simulink model "QCar2_Virtual_Car3"  (R2023a)
settings: Solver=ode1  StartTime=0.0  StopTime=inf  FixedStep=cameraStepSize/10  RelTol=1e-3  EnableMultiTasking=on
PreLoadFcn:
  | QCarSetup
values from neighbouring files (symbols this model uses):
  cameraStepSize = 3e-2    (= 0.03)    [QCarSetup.m]
  path_x = [0.826 0.836 0.846 0.856 0.866 0.876 0.886 0.896 0.906 0.916 0.926 0.936 ... (740 elements, 740x1)]    [SDTS_Paths_6_2023.mat]
  path_x2 = [-0.614 -0.604 -0.594 -0.584 -0.574 -0.564 -0.554 -0.544 -0.534 -0.524 -0.514 -0.504 ... (1090 elements, 1090x1)]    [SDTS_Paths_6_2023.mat]
  path_x3 = [-0.614 -0.603821428571 -0.593642857143 -0.583464285714 -0.573285714286 -0.563107142857 -0.552928571429 -0.54275 -0.532571428571 -0.522392857143 -0.512214285714 -0.502035714286 ... (714 elements, 714x1)]    [SDTS_Paths_6_2023.mat]
  path_x4 = [-0.614 -0.604 -0.594 -0.584 -0.574 -0.564 -0.554 -0.544 -0.534 -0.524 -0.514 -0.504 ... (1761 elements, 1761x1)]    [SDTS_Paths_6_2023.mat]
  path_x5 = [1.436 1.42588571429 1.41577142857 1.40565714286 1.39554285714 1.38542857143 1.37531428571 1.3652 1.35508571429 1.34497142857 1.33485714286 1.32474285714 ... (574 elements, 574x1)]    [SDTS_Paths_6_2023.mat]
  path_x6 = [1.436 1.42588571429 1.41577142857 1.40565714286 1.39554285714 1.38542857143 1.37531428571 1.3652 1.35508571429 1.34497142857 1.33485714286 1.32474285714 ... (1288 elements, 1288x1)]    [SDTS_Paths_6_2023.mat]
  path_y = [-1.0887 -1.0887 -1.0887 -1.0887 -1.0887 -1.0887 -1.0887 -1.0887 -1.0887 -1.0887 -1.0887 -1.0887 ... (740 elements, 740x1)]    [SDTS_Paths_6_2023.mat]
  path_y2 = [-1.0887 -1.0887 -1.0887 -1.0887 -1.0887 -1.0887 -1.0887 -1.0887 -1.0887 -1.0887 -1.0887 -1.0887 ... (1090 elements, 1090x1)]    [SDTS_Paths_6_2023.mat]
  path_y3 = [-1.0887 -1.0887 -1.0887 -1.0887 -1.0887 -1.0887 -1.0887 -1.0887 -1.0887 -1.0887 -1.0887 -1.0887 ... (714 elements, 714x1)]    [SDTS_Paths_6_2023.mat]
  path_y4 = [-1.0887 -1.0887 -1.0887 -1.0887 -1.0887 -1.0887 -1.0887 -1.0887 -1.0887 -1.0887 -1.0887 -1.0887 ... (1761 elements, 1761x1)]    [SDTS_Paths_6_2023.mat]
  path_y5 = [-0.8157 -0.8157 -0.8157 -0.8157 -0.8157 -0.8157 -0.8157 -0.8157 -0.8157 -0.8157 -0.8157 -0.8157 ... (574 elements, 574x1)]    [SDTS_Paths_6_2023.mat]
  path_y6 = [-0.8157 -0.8157 -0.8157 -0.8157 -0.8157 -0.8157 -0.8157 -0.8157 -0.8157 -0.8157 -0.8157 -0.8157 ... (1288 elements, 1288x1)]    [SDTS_Paths_6_2023.mat]
undefined symbols (not defined in the file or in its folder): DiscIntNeverNeededParam, gcbh, height, Host, JPEG, left, qc_get_step_size, top, video_display_show, width
libraries: quarc_library x71, simulink_extras x12, simulink x5
(part 3 of 5)

== system QCar2_Virtual_Car3/Speed & Steering Commander/Cross Track Controller ==
  closest point : Inport
  distance : Inport  Port=2
  xy : Inport  Port=3
  Heading : Inport  Port=4
  Cos : Trigonometry  Operator=cos
  Cos1 : Trigonometry
  Cross Product : quarc_library/Math Operations/Vectors/Cross Product
      settings: SourceProductName=QUARC Targets
  Demux : Demux  Outputs=3
  Gain3 : Gain  Gain=2
  Gain6 : Gain  Gain=10
  Integrator : Integrator  LimitOutput=on  UpperSaturationLimit=.25  LowerSaturationLimit=-.25
  Mux : Mux  Inputs=3
  Mux1 : Mux  Inputs=2
  Product3 : Product
  Saturation1 : Saturate  UpperLimit=0.25  LowerLimit=-0.25
  Sign : Signum
  Sum : Sum  Inputs=+-
  Sum2 : Sum
  steering correction : Outport
  wires:
  Sum2/1 -> steering correction/1
  distance/1 -> Product3/2
  Saturation1/1 -> Sum2/2
  Integrator/1 -> Sum2/1
  Product3/1 -> Gain6/1, Gain3/1
  Gain3/1 -> Saturation1/1
  Gain6/1 -> Integrator/1
  Sign/1 -> Product3/1
  Demux/3 -> Sign/1
  Cross Product/1 -> Demux/1
  Mux/1 -> Cross Product/1
  Mux1/1 -> Cross Product/2
  Sum/1 -> Mux1/1
  closest point/1 -> Sum/1
  xy/1 -> Sum/2
  Cos1/1 -> Mux/2
  Cos/1 -> Mux/1
  Heading/1 -> Cos/1, Cos1/1

== system QCar2_Virtual_Car3/Speed & Steering Commander/LiDAR Steering ==
  xy_command : Inport
  xy : Inport  Port=2
  heading : Inport  Port=3
  Direction Vector Generator : Subsystem
  Display1 : Display
      settings: Decimation=100
  Gain1 : Gain
  Radians to Degrees1 : simulink_extras/Transformations/Radians to Degrees
  Steering Commander : MATLAB Function  TreatAsAtomicUnit=on
  distance : Outport
  LiDAR Steering : Outport  Port=2
  wires:
  Steering Commander/1(steering) -> Gain1/1
  heading/1 -> Direction Vector Generator/3(heading)
  xy/1 -> Direction Vector Generator/2(xy)
  Radians to Degrees1/1 -> Display1/1
  Gain1/1 -> LiDAR Steering/1
  Direction Vector Generator/2(aoa) -> Steering Commander/1(aoa), Radians to Degrees1/1
  xy_command/1 -> Direction Vector Generator/1(xy_command)
  Direction Vector Generator/1(distance) -> distance/1

== system QCar2_Virtual_Car3/Speed & Steering Commander/Path Commander ==
  note: Changed the abs and the duration
  path : Inport
  xy : Inport  Port=2
  look_ahead_d : Inport  Port=3
  Constant : Constant  Value=.05
  Constant1 : Constant  Value=.5
  Data Type Conversion : DataTypeConversion  SaturateOnIntegerOverflow=off  RndMeth=Floor
  Display : Display
  "Distance  " : Scope
  Gain : Gain  Gain=[1 1 1 1 1 1]
  Less Than Threshold : Subsystem
  Multiport Switch : MultiPortSwitch  Inputs=6  DiagnosticForDefault=None  SaturateOnIntegerOverflow=off  InputSameDT=off
  Multiport Switch1 : MultiPortSwitch  Inputs=6  DiagnosticForDefault=None  SaturateOnIntegerOverflow=off  InputSameDT=off
  Multiport Switch2 : MultiPortSwitch  Inputs=6  DiagnosticForDefault=None  SaturateOnIntegerOverflow=off  InputSameDT=off
  Mux : Mux  Inputs=6
  Path 1  Look Ahead Generator : Subsystem
  Path 2  Look Ahead Generator : Subsystem
  Path 3  Look Ahead Generator : Subsystem
  Path 4  Look Ahead Generator : Subsystem
  Path 5  Look Ahead Generator : Subsystem
  Path 6  Look Ahead Generator : Subsystem
  xy_cmd : Outport
  Path_Options : Outport  Port=2
  closest point : Outport  Port=3
  distance : Outport  Port=4
  wires:
  Multiport Switch2/1 -> distance/1
  Multiport Switch1/1 -> closest point/1
  Path 6  Look Ahead Generator/2(closest_point) -> Multiport Switch1/7
  Path 5  Look Ahead Generator/2(closest_point) -> Multiport Switch1/6
  Path 4  Look Ahead Generator/2(closest_point) -> Multiport Switch1/5
  Path 3  Look Ahead Generator/2(closest_point) -> Multiport Switch1/4
  Path 2  Look Ahead Generator/2(closest_point) -> Multiport Switch1/3
  Path 1  Look Ahead Generator/2(closest_point) -> Multiport Switch1/2
  Path 6  Look Ahead Generator/3(distance) -> Mux/6, Multiport Switch2/7
  Path 5  Look Ahead Generator/3(distance) -> Mux/5, Multiport Switch2/6
  Path 6  Look Ahead Generator/1(xy_cmd) -> Multiport Switch/7
  Path 5  Look Ahead Generator/1(xy_cmd) -> Multiport Switch/6
  Data Type Conversion/1 -> Gain/1
  Gain/1 -> Path_Options/1
  Less Than Threshold/1(elapsed) -> Display/1, Data Type Conversion/1
  Constant1/1 -> Less Than Threshold/3(Duration)
  Constant/1 -> Less Than Threshold/2(Threshold)
  Mux/1 -> "Distance  "/1, Less Than Threshold/1(Signal)
  Path 4  Look Ahead Generator/3(distance) -> Mux/4, Multiport Switch2/5
  Path 3  Look Ahead Generator/3(distance) -> Mux/3, Multiport Switch2/4
  Path 2  Look Ahead Generator/3(distance) -> Mux/2, Multiport Switch2/3
  Path 1  Look Ahead Generator/3(distance) -> Mux/1, Multiport Switch2/2
  Path 4  Look Ahead Generator/1(xy_cmd) -> Multiport Switch/5
  Path 3  Look Ahead Generator/1(xy_cmd) -> Multiport Switch/4
  Multiport Switch/1 -> xy_cmd/1
  Path 2  Look Ahead Generator/1(xy_cmd) -> Multiport Switch/3
  Path 1  Look Ahead Generator/1(xy_cmd) -> Multiport Switch/2
  path/1 -> Multiport Switch/1, Multiport Switch1/1, Multiport Switch2/1
  xy/1 -> Path 1  Look Ahead Generator/1(xy), Path 2  Look Ahead Generator/1(xy), Path 3  Look Ahead Generator/1(xy), Path 4  Look Ahead Generator/1(xy), Path 5  Look Ahead Generator/1(xy), Path 6  Look Ahead Generator/1(xy)
  look_ahead_d/1 -> Path 1  Look Ahead Generator/2(look_ahead_d), Path 2  Look Ahead Generator/2(look_ahead_d), Path 3  Look Ahead Generator/2(look_ahead_d), Path 4  Look Ahead Generator/2(look_ahead_d), Path 5  Look Ahead Generator/2(look_ahead_d), Path 6  Look Ahead Generator/2(look_ahead_d)

== system QCar2_Virtual_Car3/Speed & Steering Commander/Traffic Zone 1 ==
  note: select the control variable
  xy : Inport
  speed in : Inport  Port=2
  Traffic Light : Inport  Port=3
  AND : Logic  Inputs=4  IconShape=distinctive  AllPortsSameDT=off  OutDataTypeStr=boolean
  Bias : Bias  Bias=-0.3-0.586  SaturateOnIntegerOverflow=off
  Constant13 : Constant  Value=[0.2 -0.7]+[0.586 -0.258]
  Constant14 : Constant  Value=[1 -.3] +[0.586 -0.258]
  Constant3 : Constant  Value=.1
  Demux : Demux  Outputs=2
  Demux1 : Demux  Outputs=2
  Demux2 : Demux  Outputs=2
  Gain : Gain  Gain=1/.7
  Greater Than Threshold : Subsystem
  Less Than Threshold : Subsystem
  MATLAB Function2 : MATLAB Function  TreatAsAtomicUnit=on
  Memory7 : Memory  InitialCondition=1  InheritSampleTime=on  LinearizeMemory=on  LinearizeAsDelay=on
  Saturation : Saturate  UpperLimit=1  LowerLimit=0
  "Speed " : Scope
  Speed Multi : Scope
  Traffic State : Display
  in zone : Display
  Speed Out : Outport
  wires:
  Traffic Light/1 -> MATLAB Function2/5(Traffic_Light)
  MATLAB Function2/2(Speed_Out) -> "Speed "/1, Speed Out/1
  Saturation/1 -> MATLAB Function2/3(Speed_Multi), Speed Multi/1
  AND/1 -> in zone/1, MATLAB Function2/4(In_Zone)
  speed in/1 -> MATLAB Function2/2(Speed_In)
  Memory7/1 -> MATLAB Function2/1(Previous_State)
  MATLAB Function2/1(Traffic_State) -> Traffic State/1, Memory7/1
  Gain/1 -> Saturation/1
  Bias/1 -> Gain/1
  Demux2/1 -> Bias/1
  Demux1/1 -> AND/3
  Demux1/2 -> AND/4
  Less Than Threshold/1(elapsed) -> Demux1/1
  Demux/1 -> AND/1
  Demux/2 -> AND/2
  Greater Than Threshold/1(elapsed) -> Demux/1
  Constant14/1 -> Less Than Threshold/2(Threshold)
  Constant13/1 -> Greater Than Threshold/2(Threshold)
  Constant3/1 -> Greater Than Threshold/3(Duration), Less Than Threshold/3(Duration)
  xy/1 -> Greater Than Threshold/1(Signal), Less Than Threshold/1(Signal), Demux2/1

== system QCar2_Virtual_Car3/Speed & Steering Commander/Traffic Zone 2 ==
  note: select the control variable
  xy : Inport
  speed in : Inport  Port=2
  Traffic Light : Inport  Port=3
  AND : Logic  Inputs=4  IconShape=distinctive  AllPortsSameDT=off  OutDataTypeStr=boolean
  Bias : Bias  Bias=.9-0.586  SaturateOnIntegerOverflow=off
  Constant13 : Constant  Value=[-2.2 -1]+[0.586 -0.258]
  Constant14 : Constant  Value=[-0.8 0]+[0.586 -0.258]
  Constant3 : Constant  Value=.1
  Demux : Demux  Outputs=2
  Demux1 : Demux  Outputs=2
  Demux2 : Demux  Outputs=2
  Gain : Gain  Gain=-1
  Greater Than Threshold : Subsystem
  Less Than Threshold : Subsystem
  MATLAB Function2 : MATLAB Function  TreatAsAtomicUnit=on
  Memory7 : Memory  InitialCondition=1  InheritSampleTime=on  LinearizeMemory=on  LinearizeAsDelay=on
  Saturation : Saturate  UpperLimit=1  LowerLimit=0
  "Speed " : Scope
  Speed Multi : Scope
  Traffic State : Display
  in zone : Display
  Speed Out : Outport
  wires:
  Traffic Light/1 -> MATLAB Function2/5(Traffic_Light)
  xy/1 -> Demux2/1, Less Than Threshold/1(Signal), Greater Than Threshold/1(Signal)
  Constant3/1 -> Less Than Threshold/3(Duration), Greater Than Threshold/3(Duration)
  Constant13/1 -> Greater Than Threshold/2(Threshold)
  Constant14/1 -> Less Than Threshold/2(Threshold)
  Greater Than Threshold/1(elapsed) -> Demux/1
  Demux/2 -> AND/2
  Demux/1 -> AND/1
  Less Than Threshold/1(elapsed) -> Demux1/1
  Demux1/2 -> AND/4
  Demux1/1 -> AND/3
  Demux2/1 -> Bias/1
  Bias/1 -> Gain/1
  Gain/1 -> Saturation/1
  MATLAB Function2/1(Traffic_State) -> Memory7/1, Traffic State/1
  Memory7/1 -> MATLAB Function2/1(Previous_State)
  speed in/1 -> MATLAB Function2/2(Speed_In)
  AND/1 -> MATLAB Function2/4(In_Zone), in zone/1
  Saturation/1 -> Speed Multi/1, MATLAB Function2/3(Speed_Multi)
  MATLAB Function2/2(Speed_Out) -> Speed Out/1, "Speed "/1

== system QCar2_Virtual_Car3/Speed & Steering Commander/xy signal maker ==
  In1 : Inport
  xy : Inport  Port=2
  Demux1 : Demux  Outputs=2
  Demux2 : Demux  Outputs=2
  Mux : Mux  Inputs=2
  Mux1 : Mux  Inputs=2
  Out1 : Outport
  Out2 : Outport  Port=2
  wires:
  xy/1 -> Demux2/1
  In1/1 -> Demux1/1
  Mux1/1 -> Out2/1
  Mux/1 -> Out1/1
  Demux2/2 -> Mux1/2
  Demux1/1 -> Mux/1
  Demux1/2 -> Mux1/1
  Demux2/1 -> Mux/2

== system QCar2_Virtual_Car3/Cameras/CSI Camera/Blur ==
  In1 : Inport
  Channel : quarc_library/Signal Routing/Channel  channel=0  buffer_size=1
  Image Compress : quarc_library/Image Processing/Generic/Image Compress  algorithm=JPEG  source=Internal dialog parameter  quality=quality  output_dim=-1
  Video Display : quarc_library/Multimedia/Video Display  Tag=QCar2_Virtual_Car3/Cameras/CSI Camera/Blur/Video Display  sample_time=sample_time  use_hardware=on
  wires:
  Channel/1 -> Video Display/1
  In1/1 -> Image Compress/1
  Image Compress/1 -> Channel/1

== system QCar2_Virtual_Car3/Cameras/CSI Camera/Extract Center and Slope ==
  Image : Inport
  Angle Check : Subsystem
  Center Check : Subsystem
  Constant : Constant  Value=200
  Constant1 : Constant  Value=500
  Display{1..8} (8 alike) : Display
  Gain : Gain  Gain=.085*pi/180
  Gain4 : Gain  Gain=-.05*pi/180
  MATLAB Function1 : MATLAB Function  TreatAsAtomicUnit=on
  Mux : Mux  Inputs=2
  Radians to Degrees : simulink_extras/Transformations/Radians to Degrees
  Radians to Degrees1 : simulink_extras/Transformations/Radians to Degrees
  Rate Transition : RateTransition
  Rate Transition1 : RateTransition
  Scope : Scope
  Scope3 : Scope
  Sum : Sum  Inputs=+-|
  Center Steering : Outport  VectorParamsAs1DForOutWhenUnconnected=off
  Slope Steering : Outport  Port=2  VectorParamsAs1DForOutWhenUnconnected=off
  Score : Outport  Port=3
  wires:
  Gain/1 -> Mux/2, Radians to Degrees/1, Center Steering/1
  Radians to Degrees1/1 -> Scope3/1
  Mux/1 -> Radians to Degrees1/1
  Radians to Degrees/1 -> Display2/1
  Constant/1 -> Sum/1
  Constant1/1 -> Angle Check/3(score threshold), Center Check/3(score threshold)
  MATLAB Function1/6(score) -> Center Check/1(score), Score/1, Display1/1, Scope/1, Angle Check/1(score)
  MATLAB Function1/5(b) -> Display7/1
  Center Check/1(Center Out) -> Sum/2
  Rate Transition/1 -> Gain/1
  MATLAB Function1/1(mean_x) -> Center Check/2(Center), Display8/1
  Sum/1 -> Rate Transition/1, Display3/1
  MATLAB Function1/2(mean_y) -> Display4/1
  MATLAB Function1/4(m) -> Display6/1
  Gain4/1 -> Slope Steering/1, Mux/1
  Angle Check/1(Angle Out) -> Rate Transition1/1
  MATLAB Function1/3(angle) -> Angle Check/2(Angle In), Display5/1
  Rate Transition1/1 -> Gain4/1
  Image/1 -> MATLAB Function1/1(I)

== system QCar2_Virtual_Car3/Cameras/CSI Camera/Greater Than Threshold ==
  Signal : Inport
  Threshold : Inport  Port=2
  Duration : Inport  Port=3
  Data Type Conversion : DataTypeConversion  SaturateOnIntegerOverflow=off  RndMeth=Floor
  Discrete-Time Integrator : DiscreteIntegrator  Priority=1  ExternalReset=level  SampleTime=qc_get_step_size  ICPrevOutput=DiscIntNeverNeededParam  ICPrevScaledInput=DiscIntNeverNeededParam
  Logical Operator : Logic  Operator=NOT  AllPortsSameDT=off  OutDataTypeStr=boolean
  Relational Operator : RelationalOperator  InputSameDT=off
  Relational Operator1 : RelationalOperator  InputSameDT=off
  elapsed : Outport  VectorParamsAs1DForOutWhenUnconnected=off
  time : Outport  Port=2  VectorParamsAs1DForOutWhenUnconnected=off
  wires:
  Relational Operator1/1 -> elapsed/1
  Duration/1 -> Relational Operator1/2
  Discrete-Time Integrator/1 -> time/1, Relational Operator1/1
  Logical Operator/1 -> Discrete-Time Integrator/2
  Relational Operator/1 -> Logical Operator/1, Data Type Conversion/1
  Threshold/1 -> Relational Operator/2
  Signal/1 -> Relational Operator/1
  Data Type Conversion/1 -> Discrete-Time Integrator/1

== system QCar2_Virtual_Car3/Cameras/CSI Camera/Less Than Threshold ==
  Signal : Inport
  Threshold : Inport  Port=2
  Duration : Inport  Port=3
  Data Type Conversion : DataTypeConversion  SaturateOnIntegerOverflow=off  RndMeth=Floor
  Discrete-Time Integrator : DiscreteIntegrator  Priority=1  ExternalReset=level  SampleTime=qc_get_step_size  ICPrevOutput=DiscIntNeverNeededParam  ICPrevScaledInput=DiscIntNeverNeededParam
  Logical Operator : Logic  Operator=NOT  AllPortsSameDT=off  OutDataTypeStr=boolean
  Relational Operator : RelationalOperator  Operator=<  InputSameDT=off
  Relational Operator1 : RelationalOperator  InputSameDT=off
  elapsed : Outport  VectorParamsAs1DForOutWhenUnconnected=off
  time : Outport  Port=2  VectorParamsAs1DForOutWhenUnconnected=off
  wires:
  Relational Operator1/1 -> elapsed/1
  Duration/1 -> Relational Operator1/2
  Discrete-Time Integrator/1 -> time/1, Relational Operator1/1
  Logical Operator/1 -> Discrete-Time Integrator/2
  Relational Operator/1 -> Logical Operator/1, Data Type Conversion/1
  Threshold/1 -> Relational Operator/2
  Signal/1 -> Relational Operator/1
  Data Type Conversion/1 -> Discrete-Time Integrator/1

== system QCar2_Virtual_Car3/Cameras/CSI Camera/Max 1 ==
  In1 : Inport
  Channel : quarc_library/Signal Routing/Channel  channel=1  buffer_size=1
  Image Compress : quarc_library/Image Processing/Generic/Image Compress  algorithm=JPEG  source=Internal dialog parameter  quality=quality  output_dim=-1
  Video Display : quarc_library/Multimedia/Video Display  Tag=QCar2_Virtual_Car3/Cameras/CSI Camera/Max 1/Video Display  sample_time=sample_time  use_hardware=on
  wires:
  Image Compress/1 -> Channel/1
  In1/1 -> Image Compress/1
  Channel/1 -> Video Display/1

== system QCar2_Virtual_Car3/Cameras/CSI Camera/Min 1 ==
  In1 : Inport
  Channel : quarc_library/Signal Routing/Channel  channel=2  buffer_size=1
  Image Compress : quarc_library/Image Processing/Generic/Image Compress  algorithm=JPEG  source=Internal dialog parameter  quality=quality  output_dim=-1
  Video Display : quarc_library/Multimedia/Video Display  Tag=QCar2_Virtual_Car3/Cameras/CSI Camera/Min 1/Video Display  sample_time=sample_time  use_hardware=on
  wires:
  Image Compress/1 -> Channel/1
  In1/1 -> Image Compress/1
  Channel/1 -> Video Display/1

== system QCar2_Virtual_Car3/Cameras/CSI Camera/Original Image ==
  In1 : Inport
  Channel : quarc_library/Signal Routing/Channel  channel=3  buffer_size=1
  Image Compress : quarc_library/Image Processing/Generic/Image Compress  algorithm=JPEG  source=Internal dialog parameter  quality=quality  output_dim=-1
  Video Display : quarc_library/Multimedia/Video Display  Tag=QCar2_Virtual_Car3/Cameras/CSI Camera/Original Image/Video Display  sample_time=sample_time  use_hardware=on
  wires:
  Channel/1 -> Video Display/1
  In1/1 -> Image Compress/1
  Image Compress/1 -> Channel/1

== system QCar2_Virtual_Car3/Cameras/CSI Camera/Original Segment ==
  In1 : Inport
  Channel : quarc_library/Signal Routing/Channel  channel=4  buffer_size=1
  Image Compress : quarc_library/Image Processing/Generic/Image Compress  algorithm=JPEG  source=Internal dialog parameter  quality=quality  output_dim=-1
  Video Display : quarc_library/Multimedia/Video Display  Tag=QCar2_Virtual_Car3/Cameras/CSI Camera/Original Segment/Video Display  sample_time=sample_time  use_hardware=on
  wires:
  Image Compress/1 -> Channel/1
  In1/1 -> Image Compress/1
  Channel/1 -> Video Display/1

== system QCar2_Virtual_Car3/Cameras/CSI Camera/high pass ==
  In1 : Inport
  Channel : quarc_library/Signal Routing/Channel  channel=5  buffer_size=1
  Image Compress : quarc_library/Image Processing/Generic/Image Compress  algorithm=JPEG  source=Internal dialog parameter  quality=quality  output_dim=-1
  Video Display : quarc_library/Multimedia/Video Display  Tag=QCar2_Virtual_Car3/Cameras/CSI Camera/high pass/Video Display  sample_time=sample_time  use_hardware=on
  wires:
  Channel/1 -> Video Display/1
  In1/1 -> Image Compress/1
  Image Compress/1 -> Channel/1

== system QCar2_Virtual_Car3/Cameras/CSI Camera/threshold ==
  In1 : Inport
  Channel : quarc_library/Signal Routing/Channel  channel=6  buffer_size=1
  Image Compress : quarc_library/Image Processing/Generic/Image Compress  algorithm=JPEG  source=Internal dialog parameter  quality=quality  output_dim=-1
  Video Display : quarc_library/Multimedia/Video Display  Tag=QCar2_Virtual_Car3/Cameras/CSI Camera/threshold/Video Display  sample_time=sample_time  use_hardware=on
  wires:
  Channel/1 -> Video Display/1
  In1/1 -> Image Compress/1
  Image Compress/1 -> Channel/1

== system QCar2_Virtual_Car3/Cameras/Sign Finder/Greater Than Threshold ==
  Signal : Inport
  Threshold : Inport  Port=2
  Duration : Inport  Port=3
  Data Type Conversion : DataTypeConversion  SaturateOnIntegerOverflow=off  RndMeth=Floor
  Discrete-Time Integrator : DiscreteIntegrator  Priority=1  ExternalReset=level  SampleTime=qc_get_step_size  ICPrevOutput=DiscIntNeverNeededParam  ICPrevScaledInput=DiscIntNeverNeededParam
  Logical Operator : Logic  Operator=NOT  AllPortsSameDT=off  OutDataTypeStr=boolean
  Relational Operator : RelationalOperator  InputSameDT=off
  Relational Operator1 : RelationalOperator  InputSameDT=off
  elapsed : Outport  VectorParamsAs1DForOutWhenUnconnected=off
  time : Outport  Port=2  VectorParamsAs1DForOutWhenUnconnected=off
  wires:
  Data Type Conversion/1 -> Discrete-Time Integrator/1
  Signal/1 -> Relational Operator/1
  Threshold/1 -> Relational Operator/2
  Relational Operator/1 -> Data Type Conversion/1, Logical Operator/1
  Logical Operator/1 -> Discrete-Time Integrator/2
  Discrete-Time Integrator/1 -> Relational Operator1/1, time/1
  Duration/1 -> Relational Operator1/2
  Relational Operator1/1 -> elapsed/1

== system QCar2_Virtual_Car3/Cameras/Sign Finder/Greater Than Threshold1 ==
  Signal : Inport
  Threshold : Inport  Port=2
  Duration : Inport  Port=3
  Data Type Conversion : DataTypeConversion  SaturateOnIntegerOverflow=off  RndMeth=Floor
  Discrete-Time Integrator : DiscreteIntegrator  Priority=1  ExternalReset=level  SampleTime=qc_get_step_size  ICPrevOutput=DiscIntNeverNeededParam  ICPrevScaledInput=DiscIntNeverNeededParam
  Logical Operator : Logic  Operator=NOT  AllPortsSameDT=off  OutDataTypeStr=boolean
  Relational Operator : RelationalOperator  InputSameDT=off
  Relational Operator1 : RelationalOperator  InputSameDT=off
  elapsed : Outport  VectorParamsAs1DForOutWhenUnconnected=off
  time : Outport  Port=2  VectorParamsAs1DForOutWhenUnconnected=off
  wires:
  Relational Operator1/1 -> elapsed/1
  Duration/1 -> Relational Operator1/2
  Discrete-Time Integrator/1 -> time/1, Relational Operator1/1
  Logical Operator/1 -> Discrete-Time Integrator/2
  Relational Operator/1 -> Logical Operator/1, Data Type Conversion/1
  Threshold/1 -> Relational Operator/2
  Signal/1 -> Relational Operator/1
  Data Type Conversion/1 -> Discrete-Time Integrator/1

== system QCar2_Virtual_Car3/QCar/To//From Simulation/RGB ==
  In1 : Inport
  Enable : EnablePort  StatesWhenEnabling=reset
  Image Decompress : quarc_library/Image Processing/Generic/Image Decompress  algorithm=JPEG  resolution=custom  width=820  height=410  output_format=MATLAB RGB (HxWx3)  data_type=uint8
      settings: AttributesFormatString=(%<algorithm>)  SourceProductName=QUARC Targets
  RGB : Outport  VectorParamsAs1DForOutWhenUnconnected=off
  wires:
  Image Decompress/1 -> RGB/1
  In1/1 -> Image Decompress/1

== system QCar2_Virtual_Car3/QCar/To//From Simulation/RGB1 ==
  In1 : Inport
  Enable : EnablePort  StatesWhenEnabling=reset
  Image Decompress : quarc_library/Image Processing/Generic/Image Decompress  algorithm=JPEG  resolution=custom  width=820  height=410  output_format=MATLAB RGB (HxWx3)  data_type=uint8
      settings: AttributesFormatString=(%<algorithm>)  SourceProductName=QUARC Targets
  RGB : Outport  VectorParamsAs1DForOutWhenUnconnected=off
  wires:
  Image Decompress/1 -> RGB/1
  In1/1 -> Image Decompress/1

== system QCar2_Virtual_Car3/QCar/To//From Simulation/RGB2 ==
  In1 : Inport
  Enable : EnablePort  StatesWhenEnabling=reset
  Image Decompress : quarc_library/Image Processing/Generic/Image Decompress  algorithm=JPEG  resolution=custom  width=820  height=410  output_format=MATLAB RGB (HxWx3)  data_type=uint8
      settings: AttributesFormatString=(%<algorithm>)  SourceProductName=QUARC Targets
  RGB : Outport  VectorParamsAs1DForOutWhenUnconnected=off
  wires:
  Image Decompress/1 -> RGB/1
  In1/1 -> Image Decompress/1

== system QCar2_Virtual_Car3/QCar/To//From Simulation/RGB3 ==
  In1 : Inport
  Enable : EnablePort  StatesWhenEnabling=reset
  Image Decompress : quarc_library/Image Processing/Generic/Image Decompress  algorithm=JPEG  resolution=custom  width=820  height=410  output_format=MATLAB RGB (HxWx3)  data_type=uint8
      settings: AttributesFormatString=(%<algorithm>)  SourceProductName=QUARC Targets
  RGB : Outport  VectorParamsAs1DForOutWhenUnconnected=off
  wires:
  Image Decompress/1 -> RGB/1
  In1/1 -> Image Decompress/1

== system QCar2_Virtual_Car3/QCar/To//From Simulation/RGB4 ==
  In1 : Inport
  Enable : EnablePort  StatesWhenEnabling=reset
  Image Decompress : quarc_library/Image Processing/Generic/Image Decompress  algorithm=JPEG  resolution=640 x 480  width=640  height=480  output_format=MATLAB RGB (HxWx3)  data_type=uint8
      settings: AttributesFormatString=(%<algorithm>)  SourceProductName=QUARC Targets
  RGB : Outport  VectorParamsAs1DForOutWhenUnconnected=off
  wires:
  Image Decompress/1 -> RGB/1
  In1/1 -> Image Decompress/1

== system QCar2_Virtual_Car3/QCar/To//From Simulation/RGB5 ==
  In1 : Inport
  Enable : EnablePort  StatesWhenEnabling=reset
  Image Decompress : quarc_library/Image Processing/Generic/Image Decompress  algorithm=JPEG  resolution=640 x 480  width=640  height=480  output_format=MATLAB RGB (HxWx3)  data_type=uint8
      settings: AttributesFormatString=(%<algorithm>)  SourceProductName=QUARC Targets
  RGB : Outport  VectorParamsAs1DForOutWhenUnconnected=off
  wires:
  Image Decompress/1 -> RGB/1
  In1/1 -> Image Decompress/1

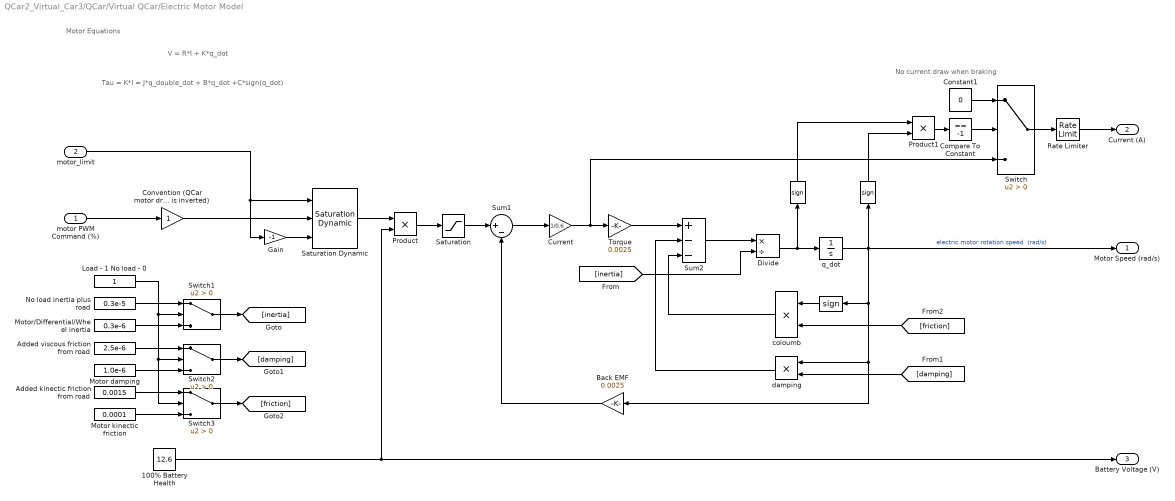
== system QCar2_Virtual_Car3/QCar/Virtual QCar/Electric Motor Model ==
  note: No current draw when braking
  note: Motor Equations
  note: Tau = K*I = J*q_double_dot + B*q_dot +C*sign(q_dot)
  note: V = R*I + K*q_dot
  motor PWM Command (%) : Inport
  motor_limit : Inport  Port=2
  " " : Signum
  "  " : Signum
  "   " : Signum
  100% Battery Health : Constant  Value=12.6
  Added kinectic friction from road : Constant  Value=0.0015
  Added viscous friction from road : Constant  Value=2.5e-6
  Back EMF : Gain  Gain=0.0025
  Compare To Constant : simulink/Logic and Bit Operations/Compare To Constant  relop===  const=-1  OutDataTypeStr=boolean
  Constant1 : Constant  Value=0
  Convention (QCar motor drive is inverted) : Gain
  Current : Gain  Gain=1/0.6
  Divide : Product  Inputs=*/
  Gain : Gain  Gain=-1
  Load - 1 No load - 0 : Constant
  Motor damping : Constant  Value=1.0e-6
  Motor kinectic friction : Constant  Value=0.0001
  Motor/Differential/Wheel inertia : Constant  Value=0.3e-6
  No load inertia plus road : Constant  Value=0.3e-5
  Product : Product
  Product1 : Product
  Rate Limiter : RateLimiter  RisingSlewLimit=1*10  FallingSlewLimit=-1*10  SampleTimeMode=inherited
  Saturation : Saturate  UpperLimit=12.6  LowerLimit=-12.6
  Saturation Dynamic : simulink/Discontinuities/Saturation Dynamic  OutMin=[]  OutMax=[]  OutDataTypeStr=Inherit: Same as second input  OutDataType=fixdt(1, 16)  OutScaling=2^-10  DoSatur=off
  Sum1 : Sum  Inputs=|+-
  Sum2 : Sum  Inputs=+--
  Switch{,1..3} (4 alike) : Switch  Criteria=u2 > Threshold  SaturateOnIntegerOverflow=off  InputSameDT=off
  Torque : Gain  Gain=0.0025
  coloumb : Product
  damping : Product
  q_dot : Integrator
  Motor Speed (rad/s) : Outport
  Current (A) : Outport  Port=2
  Battery Voltage (V) : Outport  Port=3
  wires:
  Back EMF/1 -> Sum1/2
  q_dot/1 -> "  "/1, " "/1, Back EMF/1, damping/1, Motor Speed (rad/s)/1  "electric motor rotation speed  (rad/s)"
  coloumb/1 -> Sum2/3
  Sum1/1 -> Current/1
  100% Battery Health/1 -> Product/2, Battery Voltage (V)/1
  Sum2/1 -> Divide/1
  Torque/1 -> Sum2/1
  "  "/1 -> Product1/2
  damping/1 -> Sum2/2
  Divide/1 -> q_dot/1, "   "/1
  Product/1 -> Saturation/1
  motor PWM Command (%)/1 -> Convention (QCar motor drive is inverted)/1
  Saturation Dynamic/1 -> Product/1
  motor_limit/1 -> Gain/1, Saturation Dynamic/1
  Gain/1 -> Saturation Dynamic/3
  Convention (QCar motor drive is inverted)/1 -> Saturation Dynamic/2
  [damping] -> damping/2
  [friction] -> coloumb/2
  Current/1 -> Torque/1, Switch/3
  Saturation/1 -> Sum1/1
  "   "/1 -> Product1/1
  Product1/1 -> Compare To Constant/1
  Compare To Constant/1 -> Switch/2
  Constant1/1 -> Switch/1
  Switch/1 -> Rate Limiter/1
  Rate Limiter/1 -> Current (A)/1
  Load - 1 No load - 0/1 -> Switch2/2, Switch3/2, Switch1/2
  No load inertia plus road/1 -> Switch1/1
  Motor/Differential/Wheel inertia/1 -> Switch1/3
  Added viscous friction from road/1 -> Switch2/1
  Motor damping/1 -> Switch2/3
  Added kinectic friction from road/1 -> Switch3/1
  Motor kinectic friction/1 -> Switch3/3
  Switch1/1 -> [inertia]
  Switch2/1 -> [damping]
  Switch3/1 -> [friction]
  [inertia] -> Divide/2
  " "/1 -> coloumb/1

== system QCar2_Virtual_Car3/QCar/Virtual QCar/LED Logic ==
  note: Headlights, Brakes, Left, Right
  Speed : Inport
  Throttle : Inport  Port=2
  Headlights : Inport  Port=3
  Steering : Inport  Port=4
  " Brake" : Logic  Operator=OR  IconShape=distinctive  AllPortsSameDT=off  OutDataTypeStr=boolean
  AND : Logic  IconShape=distinctive  AllPortsSameDT=off  OutDataTypeStr=boolean
  Constant1 : Constant  Value=20
  Constant2 : Constant  Value=.1
  Constant3 : Constant  Value=0
  Constant4 : Constant  Value=.1
  Constant5 : Constant  Value=0
  Constant6 : Constant  Value=.2
  Constant7 : Constant  Value=.01
  Constant8 : Constant  Value=.1
  Gain : Gain  Gain=-1
  Gain1 : Gain  Gain=-1
  Greater Than Threshold1 : Subsystem
  Left Threshold : Subsystem
  Less Than Threshold1 : Subsystem
  Less Than Threshold2 : Subsystem
  Less Than Threshold3 : Subsystem
  MATLAB Function : MATLAB Function  TreatAsAtomicUnit=on
  Pulse Generator : DiscretePulseGenerator  Period=500  PulseWidth=250  SampleTime=qc_get_step_size
  Radians to Degrees : simulink_extras/Transformations/Radians to Degrees
  Right Threshold : Subsystem
  LEDs : Outport
  wires:
  Gain1/1 -> Greater Than Threshold1/2(Threshold)
  AND/1 -> " Brake"/2
  Greater Than Threshold1/1(elapsed) -> AND/2
  Less Than Threshold3/1(elapsed) -> AND/1
  Constant8/1 -> Less Than Threshold3/2(Threshold), Gain1/1
  Constant7/1 -> Greater Than Threshold1/3(Duration), Less Than Threshold3/3(Duration)
  Less Than Threshold2/1(elapsed) -> " Brake"/1
  Constant6/1 -> Less Than Threshold2/3(Duration)
  Constant5/1 -> Less Than Threshold2/2(Threshold)
  Throttle/1 -> Less Than Threshold2/1(Signal)
  Constant4/1 -> Less Than Threshold1/3(Duration)
  Constant3/1 -> Less Than Threshold1/2(Threshold)
  Speed/1 -> Less Than Threshold1/1(Signal), Greater Than Threshold1/1(Signal), Less Than Threshold3/1(Signal)
  Gain/1 -> Right Threshold/2(Threshold)
  Constant2/1 -> Left Threshold/3(Duration), Right Threshold/3(Duration)
  Constant1/1 -> Left Threshold/2(Threshold), Gain/1
  Radians to Degrees/1 -> Left Threshold/1(Signal), Right Threshold/1(Signal)
  Steering/1 -> Radians to Degrees/1
  MATLAB Function/1(lights) -> LEDs/1
  Pulse Generator/1 -> MATLAB Function/6(pulse)
  Headlights/1 -> MATLAB Function/1(headlights)
  " Brake"/1 -> MATLAB Function/2(breaklights)
  Left Threshold/1(elapsed) -> MATLAB Function/4(leftTurn)
  Right Threshold/1(elapsed) -> MATLAB Function/5(rightTurn)

== system QCar2_Virtual_Car3/QCar/Virtual QCar/basicSpeedEstimation ==
  note: Estimate car speed from motor encoder counts rate
  note: v = 2*pi*r * omega (if omega is in rot/s)
      | v = r * omega (if omega is in rad/s)
      | r = 0.0342 m
  note: (Diff. pinion*pinion)/(Spur*Diff. spur)
  note: speedEstimation Module:
      |
      | This subsystem converts the motor speed measurements in counts/s to a useful longitudinal car speed in m/s.
      |
      | Inputs:
      | motorSpeed (counts/s) n/a : Drive motor speed measured using an encoder
      |
      | Outputs:
      | longitudinalCarSpeed (m/s) n/a : The platform's longitudinal speed (along the front-rear axis direction)
  motorSpeed (rad/s) : Inport
  gear ratios : Gain  Gain=(13*19)/(70*37)
  to rot/s : Gain
  wheel radius : Gain  Gain=0.0342
  longitudinalCarSpeed (m/s) : Outport  VectorParamsAs1DForOutWhenUnconnected=off
  wires:
  motorSpeed (rad/s)/1 -> to rot/s/1  "motor speed (rot/s)"
  wheel radius/1 -> longitudinalCarSpeed (m/s)/1  "wheel speed (m/s)"
  gear ratios/1 -> wheel radius/1  "shaft speed (rots/s)"
  to rot/s/1 -> gear ratios/1  "wheel speed (m/s)"

== system QCar2_Virtual_Car3/QCar/Virtual QCar/speedController ==
  note: Feedforward
  note: Feedback
  arm (0,1) : Inport
  desiredSpeed (m/s) : Inport  Port=2
  measuredSpeed (m/s) : Inport  Port=3
  Add : Sum
  Add1 : Sum
  Compare To Zero : simulink/Logic and Bit Operations/Compare To Zero  relop===  OutDataTypeStr=boolean
  Integrator1 : Integrator  ExternalReset=either  LimitOutput=on  UpperSaturationLimit=0.4  LowerSaturationLimit=-0.4
  Kff (% / m/s) : Gain  Gain=0.1
  "Ki (% / m) " : Gain  Gain=.5
  Kp (% / m/s) : Gain  Gain=.5
  Multiply : Product
  Multiply1 : Product
  Multiply2 : Product
  Speed_Tracking : Scope  NumInputPorts=2
  Sum : Sum  Inputs=|+-
  command saturation : Saturate  UpperLimit=5  LowerLimit=-5
  PWM Cmd : Outport  VectorParamsAs1DForOutWhenUnconnected=off
  wires:
  command saturation/1 -> Multiply1/1  "desired"
  arm (0,1)/1 -> Multiply1/2, Multiply/2, Multiply2/2
  measuredSpeed (m/s)/1 -> Multiply/1  "meas"
  Multiply/1 -> Sum/2, Speed_Tracking/2  "measured"
  Add/1 -> Add1/2
  Add1/1 -> Multiply2/1  "%"
  Multiply1/1 -> Compare To Zero/1, Sum/1, Kff (% / m/s)/1, Speed_Tracking/1  "desired"
  Integrator1/1 -> Add/2
  Kp (% / m/s)/1 -> Add/1
  Compare To Zero/1 -> Integrator1/2
  Kff (% / m/s)/1 -> Add1/1
  Sum/1 -> "Ki (% / m) "/1, Kp (% / m/s)/1
  "Ki (% / m) "/1 -> Integrator1/1
  Multiply2/1 -> PWM Cmd/1  "pwm duty cycle"
  desiredSpeed (m/s)/1 -> command saturation/1

== system QCar2_Virtual_Car3/Randomizer/Subsystem1/RisingEdge ==
  Input : Inport
  Logical Operator1 : Logic  AllPortsSameDT=off
  Logical Operator2 : Logic  Operator=NOT  AllPortsSameDT=off
  Memory : Memory  InheritSampleTime=on  LinearizeMemory=on
  RisingEdgeTrigger : Outport  VectorParamsAs1DForOutWhenUnconnected=off
  wires:
  Input/1 -> Memory/1, Logical Operator1/1
  Memory/1 -> Logical Operator2/1
  Logical Operator2/1 -> Logical Operator1/2
  Logical Operator1/1 -> RisingEdgeTrigger/1

== system QCar2_Virtual_Car3/Speed & Steering Commander/LiDAR Steering/Direction Vector Generator ==
  xy_command : Inport
  xy : Inport  Port=2
  heading : Inport  Port=3
  Demux : Demux  Outputs=2
  Display2 : Display
      settings: Decimation=100
  Display5 : Display
      settings: Decimation=100
  Display8 : Display
      settings: Decimation=100
  Radians to Degrees1 : simulink_extras/Transformations/Radians to Degrees
  Radians to Degrees3 : simulink_extras/Transformations/Radians to Degrees
  Signed Sqrt : Sqrt
  Square : Math  Operator=square
  Sum : Sum  Inputs=+-
  Sum1 : Sum  Inputs=+
  Sum3 : Sum  Inputs=+-
  Trigonometric Function : Trigonometry  Operator=atan2
  distance : Outport
  aoa : Outport  Port=2
  wires:
  xy_command/1 -> Sum/1
  Demux/1 -> Trigonometric Function/2
  Trigonometric Function/1 -> Sum3/1, Radians to Degrees1/1
  Square/1 -> Sum1/1
  Signed Sqrt/1 -> Display8/1, distance/1
  xy/1 -> Sum/2
  Sum3/1 -> Radians to Degrees3/1, aoa/1
  Sum1/1 -> Signed Sqrt/1
  Demux/2 -> Trigonometric Function/1
  Radians to Degrees1/1 -> Display5/1
  Radians to Degrees3/1 -> Display2/1
  Sum/1 -> Square/1, Demux/1
  heading/1 -> Sum3/2

== system QCar2_Virtual_Car3/Speed & Steering Commander/Path Commander/Less Than Threshold ==
  Signal : Inport
  Threshold : Inport  Port=2
  Duration : Inport  Port=3
  Data Type Conversion : DataTypeConversion  SaturateOnIntegerOverflow=off  RndMeth=Floor
  Discrete-Time Integrator : DiscreteIntegrator  Priority=1  ExternalReset=level  SampleTime=qc_get_step_size  ICPrevOutput=DiscIntNeverNeededParam  ICPrevScaledInput=DiscIntNeverNeededParam
  Logical Operator : Logic  Operator=NOT  AllPortsSameDT=off  OutDataTypeStr=boolean
  Relational Operator : RelationalOperator  Operator=<  InputSameDT=off
  Relational Operator1 : RelationalOperator  InputSameDT=off
  elapsed : Outport  VectorParamsAs1DForOutWhenUnconnected=off
  time : Outport  Port=2  VectorParamsAs1DForOutWhenUnconnected=off
  wires:
  Relational Operator1/1 -> elapsed/1
  Duration/1 -> Relational Operator1/2
  Discrete-Time Integrator/1 -> time/1, Relational Operator1/1
  Logical Operator/1 -> Discrete-Time Integrator/2
  Relational Operator/1 -> Logical Operator/1, Data Type Conversion/1
  Threshold/1 -> Relational Operator/2
  Signal/1 -> Relational Operator/1
  Data Type Conversion/1 -> Discrete-Time Integrator/1

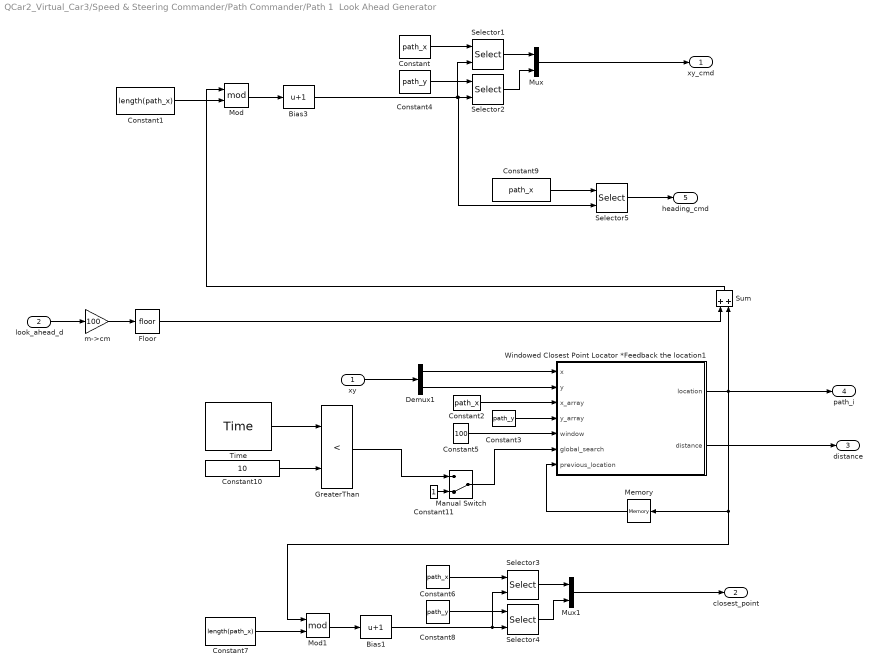
== system QCar2_Virtual_Car3/Speed & Steering Commander/Path Commander/Path 1  Look Ahead Generator ==
  xy : Inport
  look_ahead_d : Inport  Port=2
  Bias1 : Bias  Bias=1  SaturateOnIntegerOverflow=off
  Bias3 : Bias  Bias=1  SaturateOnIntegerOverflow=off
  Constant{,2,6,9} (4 alike) : Constant  Value=path_x
  Constant1 : Constant  Value=length(path_x)
  Constant10 : Constant  Value=10
  Constant11 : Constant
  Constant3 : Constant  Value=path_y
  Constant4 : Constant  Value=path_y
  Constant5 : Constant  Value=100
  Constant7 : Constant  Value=length(path_x)
  Constant8 : Constant  Value=path_y
  Demux1 : Demux  Outputs=2
  Floor : Rounding
  GreaterThan : RelationalOperator  Operator=<  OutDataTypeStr=boolean  RndMeth=Simplest  InputSameDT=off
  Manual Switch : ManualSwitch  CurrentSetting=0
  Memory : Memory  InitialCondition=1  InheritSampleTime=on  LinearizeMemory=on  LinearizeAsDelay=on
  Mod : Math  Operator=mod
  Mod1 : Math  Operator=mod
  Mux : Mux  Inputs=2
  Mux1 : Mux  Inputs=2
  Selector{1..5} (5 alike) : Selector  InputPortWidth=length(path_x)  IndexOptions=Index vector (port)  Indices=[1 3]  OutputSizes=1
  Sum : Sum
  Time : quarc_library/Sources/Time/Time  time_source=Wall clock  sample_time=qc_get_step_size
  Windowed Closest Point Locator *Feedback the location1 : MATLAB Function  TreatAsAtomicUnit=on
  m->cm : Gain  Gain=100
  xy_cmd : Outport
  closest_point : Outport  Port=2
  distance : Outport  Port=3
  path_i : Outport  Port=4
  heading_cmd : Outport  Port=5
  wires:
  GreaterThan/1 -> Manual Switch/1
  Manual Switch/1 -> Windowed Closest Point Locator *Feedback the location1/6(global_search)
  Constant11/1 -> Manual Switch/2
  Memory/1 -> Windowed Closest Point Locator *Feedback the location1/7(previous_location)
  Constant5/1 -> Windowed Closest Point Locator *Feedback the location1/5(window)
  Constant10/1 -> GreaterThan/2
  Time/1 -> GreaterThan/1
  Selector5/1 -> heading_cmd/1
  Constant9/1 -> Selector5/1
  Bias3/1 -> Selector2/2, Selector5/2, Selector1/2
  Windowed Closest Point Locator *Feedback the location1/1(location) -> Memory/1, Mod1/1, path_i/1, Sum/2
  Selector3/1 -> Mux1/1
  Constant8/1 -> Selector4/1
  Constant7/1 -> Mod1/2
  Mod1/1 -> Bias1/1
  Constant6/1 -> Selector3/1
  Selector4/1 -> Mux1/2
  Bias1/1 -> Selector4/2, Selector3/2
  Mux1/1 -> closest_point/1
  Windowed Closest Point Locator *Feedback the location1/2(distance) -> distance/1
  Selector2/1 -> Mux/2
  Mux/1 -> xy_cmd/1
  Constant4/1 -> Selector2/1
  Selector1/1 -> Mux/1
  Constant/1 -> Selector1/1
  Floor/1 -> Sum/1
  m->cm/1 -> Floor/1
  look_ahead_d/1 -> m->cm/1
  xy/1 -> Demux1/1
  Mod/1 -> Bias3/1
  Demux1/2 -> Windowed Closest Point Locator *Feedback the location1/2(y)
  Sum/1 -> Mod/1
  Constant1/1 -> Mod/2
  Constant3/1 -> Windowed Closest Point Locator *Feedback the location1/4(y_array)
  Constant2/1 -> Windowed Closest Point Locator *Feedback the location1/3(x_array)
  Demux1/1 -> Windowed Closest Point Locator *Feedback the location1/1(x)

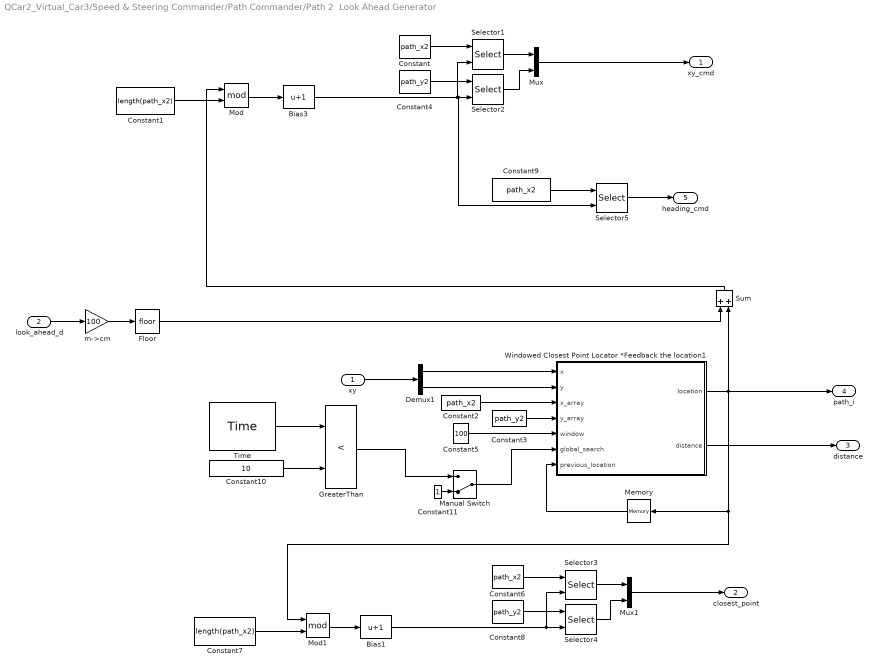
== system QCar2_Virtual_Car3/Speed & Steering Commander/Path Commander/Path 2  Look Ahead Generator ==
  xy : Inport
  look_ahead_d : Inport  Port=2
  Bias1 : Bias  Bias=1  SaturateOnIntegerOverflow=off
  Bias3 : Bias  Bias=1  SaturateOnIntegerOverflow=off
  Constant{,2,6,9} (4 alike) : Constant  Value=path_x2
  Constant1 : Constant  Value=length(path_x2)
  Constant10 : Constant  Value=10
  Constant11 : Constant
  Constant3 : Constant  Value=path_y2
  Constant4 : Constant  Value=path_y2
  Constant5 : Constant  Value=100
  Constant7 : Constant  Value=length(path_x2)
  Constant8 : Constant  Value=path_y2
  Demux1 : Demux  Outputs=2
  Floor : Rounding
  GreaterThan : RelationalOperator  Operator=<  OutDataTypeStr=boolean  RndMeth=Simplest  InputSameDT=off
  Manual Switch : ManualSwitch  CurrentSetting=0
  Memory : Memory  InitialCondition=1  InheritSampleTime=on  LinearizeMemory=on  LinearizeAsDelay=on
  Mod : Math  Operator=mod
  Mod1 : Math  Operator=mod
  Mux : Mux  Inputs=2
  Mux1 : Mux  Inputs=2
  Selector{1..5} (5 alike) : Selector  InputPortWidth=length(path_x2)  IndexOptions=Index vector (port)  Indices=[1 3]  OutputSizes=1
  Sum : Sum
  Time : quarc_library/Sources/Time/Time  time_source=Wall clock  sample_time=qc_get_step_size
  Windowed Closest Point Locator *Feedback the location1 : MATLAB Function  TreatAsAtomicUnit=on
  m->cm : Gain  Gain=100
  xy_cmd : Outport
  closest_point : Outport  Port=2
  distance : Outport  Port=3
  path_i : Outport  Port=4
  heading_cmd : Outport  Port=5
  wires:
  GreaterThan/1 -> Manual Switch/1
  Constant11/1 -> Manual Switch/2
  Manual Switch/1 -> Windowed Closest Point Locator *Feedback the location1/6(global_search)
  Constant10/1 -> GreaterThan/2
  Time/1 -> GreaterThan/1
  Mux1/1 -> closest_point/1
  Selector4/1 -> Mux1/2
  Bias1/1 -> Selector4/2, Selector3/2
  Constant6/1 -> Selector3/1
  Selector3/1 -> Mux1/1
  Constant8/1 -> Selector4/1
  Demux1/1 -> Windowed Closest Point Locator *Feedback the location1/1(x)
  Constant2/1 -> Windowed Closest Point Locator *Feedback the location1/3(x_array)
  Constant3/1 -> Windowed Closest Point Locator *Feedback the location1/4(y_array)
  Constant1/1 -> Mod/2
  Sum/1 -> Mod/1
  Demux1/2 -> Windowed Closest Point Locator *Feedback the location1/2(y)
  Mod/1 -> Bias3/1
  xy/1 -> Demux1/1
  look_ahead_d/1 -> m->cm/1
  m->cm/1 -> Floor/1
  Floor/1 -> Sum/1
  Constant/1 -> Selector1/1
  Selector1/1 -> Mux/1
  Constant4/1 -> Selector2/1
  Mux/1 -> xy_cmd/1
  Selector2/1 -> Mux/2
  Windowed Closest Point Locator *Feedback the location1/2(distance) -> distance/1
  Mod1/1 -> Bias1/1
  Constant7/1 -> Mod1/2
  Windowed Closest Point Locator *Feedback the location1/1(location) -> Sum/2, path_i/1, Mod1/1, Memory/1
  Bias3/1 -> Selector1/2, Selector5/2, Selector2/2
  Constant9/1 -> Selector5/1
  Selector5/1 -> heading_cmd/1
  Constant5/1 -> Windowed Closest Point Locator *Feedback the location1/5(window)
  Memory/1 -> Windowed Closest Point Locator *Feedback the location1/7(previous_location)

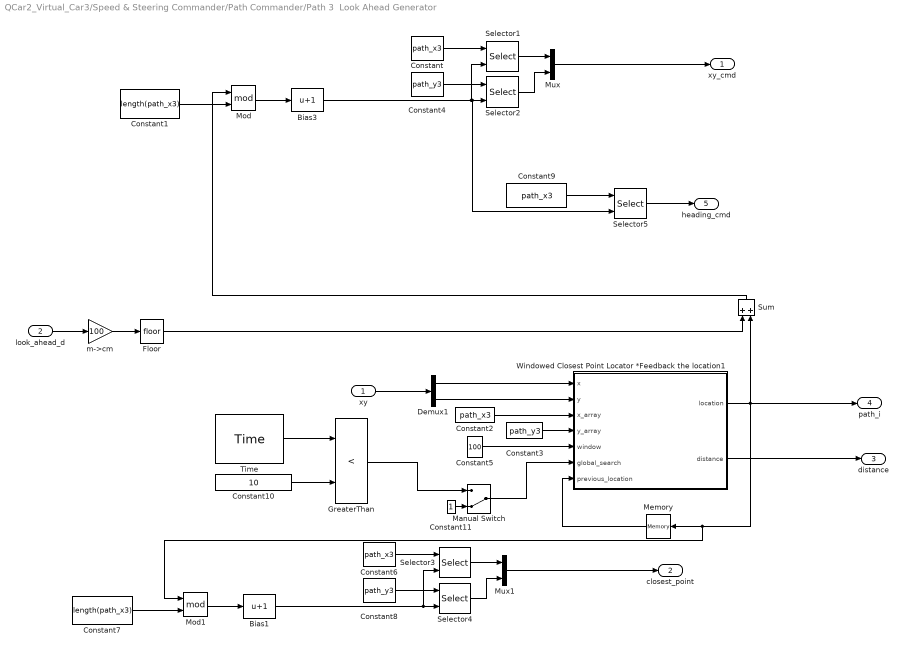
== system QCar2_Virtual_Car3/Speed & Steering Commander/Path Commander/Path 3  Look Ahead Generator ==
  xy : Inport
  look_ahead_d : Inport  Port=2
  Bias1 : Bias  Bias=1  SaturateOnIntegerOverflow=off
  Bias3 : Bias  Bias=1  SaturateOnIntegerOverflow=off
  Constant{,2,6,9} (4 alike) : Constant  Value=path_x3
  Constant1 : Constant  Value=length(path_x3)
  Constant10 : Constant  Value=10
  Constant11 : Constant
  Constant3 : Constant  Value=path_y3
  Constant4 : Constant  Value=path_y3
  Constant5 : Constant  Value=100
  Constant7 : Constant  Value=length(path_x3)
  Constant8 : Constant  Value=path_y3
  Demux1 : Demux  Outputs=2
  Floor : Rounding
  GreaterThan : RelationalOperator  Operator=<  OutDataTypeStr=boolean  RndMeth=Simplest  InputSameDT=off
  Manual Switch : ManualSwitch  CurrentSetting=0
  Memory : Memory  InitialCondition=1  InheritSampleTime=on  LinearizeMemory=on  LinearizeAsDelay=on
  Mod : Math  Operator=mod
  Mod1 : Math  Operator=mod
  Mux : Mux  Inputs=2
  Mux1 : Mux  Inputs=2
  Selector{1..5} (5 alike) : Selector  InputPortWidth=length(path_x3)  IndexOptions=Index vector (port)  Indices=[1 3]  OutputSizes=1
  Sum : Sum
  Time : quarc_library/Sources/Time/Time  time_source=Wall clock  sample_time=qc_get_step_size
  Windowed Closest Point Locator *Feedback the location1 : MATLAB Function  TreatAsAtomicUnit=on
  m->cm : Gain  Gain=100
  xy_cmd : Outport
  closest_point : Outport  Port=2
  distance : Outport  Port=3
  path_i : Outport  Port=4
  heading_cmd : Outport  Port=5
  wires:
  GreaterThan/1 -> Manual Switch/1
  Constant11/1 -> Manual Switch/2
  Manual Switch/1 -> Windowed Closest Point Locator *Feedback the location1/6(global_search)
  Constant10/1 -> GreaterThan/2
  Time/1 -> GreaterThan/1
  Bias1/1 -> Selector4/2, Selector3/2
  Constant7/1 -> Mod1/2
  Constant6/1 -> Selector3/1
  Mod1/1 -> Bias1/1
  Windowed Closest Point Locator *Feedback the location1/1(location) -> Memory/1, Mod1/1, path_i/1, Sum/2
  Constant8/1 -> Selector4/1
  Mux1/1 -> closest_point/1
  Selector3/1 -> Mux1/1
  Selector4/1 -> Mux1/2
  Memory/1 -> Windowed Closest Point Locator *Feedback the location1/7(previous_location)
  Constant5/1 -> Windowed Closest Point Locator *Feedback the location1/5(window)
  Selector5/1 -> heading_cmd/1
  Constant9/1 -> Selector5/1
  Bias3/1 -> Selector2/2, Selector5/2, Selector1/2
  Windowed Closest Point Locator *Feedback the location1/2(distance) -> distance/1
  Selector2/1 -> Mux/2
  Mux/1 -> xy_cmd/1
  Constant4/1 -> Selector2/1
  Selector1/1 -> Mux/1
  Constant/1 -> Selector1/1
  Floor/1 -> Sum/1
  m->cm/1 -> Floor/1
  look_ahead_d/1 -> m->cm/1
  xy/1 -> Demux1/1
  Mod/1 -> Bias3/1
  Demux1/2 -> Windowed Closest Point Locator *Feedback the location1/2(y)
  Sum/1 -> Mod/1
  Constant1/1 -> Mod/2
  Constant3/1 -> Windowed Closest Point Locator *Feedback the location1/4(y_array)
  Constant2/1 -> Windowed Closest Point Locator *Feedback the location1/3(x_array)
  Demux1/1 -> Windowed Closest Point Locator *Feedback the location1/1(x)

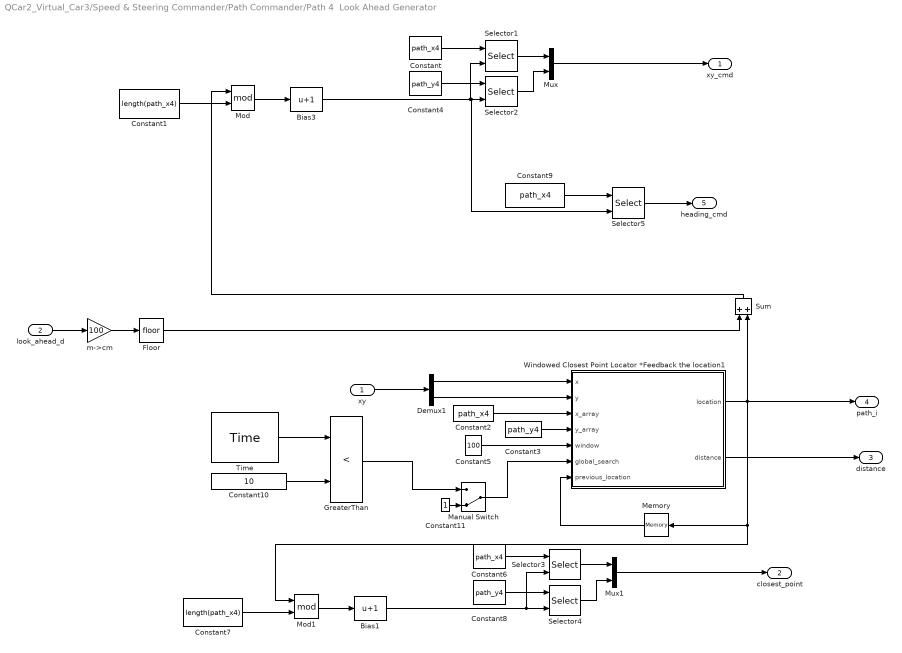
== system QCar2_Virtual_Car3/Speed & Steering Commander/Path Commander/Path 4  Look Ahead Generator ==
  xy : Inport
  look_ahead_d : Inport  Port=2
  Bias1 : Bias  Bias=1  SaturateOnIntegerOverflow=off
  Bias3 : Bias  Bias=1  SaturateOnIntegerOverflow=off
  Constant{,2,6,9} (4 alike) : Constant  Value=path_x4
  Constant1 : Constant  Value=length(path_x4)
  Constant10 : Constant  Value=10
  Constant11 : Constant
  Constant3 : Constant  Value=path_y4
  Constant4 : Constant  Value=path_y4
  Constant5 : Constant  Value=100
  Constant7 : Constant  Value=length(path_x4)
  Constant8 : Constant  Value=path_y4
  Demux1 : Demux  Outputs=2
  Floor : Rounding
  GreaterThan : RelationalOperator  Operator=<  OutDataTypeStr=boolean  RndMeth=Simplest  InputSameDT=off
  Manual Switch : ManualSwitch  CurrentSetting=0
  Memory : Memory  InitialCondition=1  InheritSampleTime=on  LinearizeMemory=on  LinearizeAsDelay=on
  Mod : Math  Operator=mod
  Mod1 : Math  Operator=mod
  Mux : Mux  Inputs=2
  Mux1 : Mux  Inputs=2
  Selector{1..5} (5 alike) : Selector  InputPortWidth=length(path_x4)  IndexOptions=Index vector (port)  Indices=[1 3]  OutputSizes=1
  Sum : Sum
  Time : quarc_library/Sources/Time/Time  time_source=Wall clock  sample_time=qc_get_step_size
  Windowed Closest Point Locator *Feedback the location1 : MATLAB Function  TreatAsAtomicUnit=on
  m->cm : Gain  Gain=100
  xy_cmd : Outport
  closest_point : Outport  Port=2
  distance : Outport  Port=3
  path_i : Outport  Port=4
  heading_cmd : Outport  Port=5
  wires:
  GreaterThan/1 -> Manual Switch/1
  Constant11/1 -> Manual Switch/2
  Manual Switch/1 -> Windowed Closest Point Locator *Feedback the location1/6(global_search)
  Constant10/1 -> GreaterThan/2
  Time/1 -> GreaterThan/1
  Constant6/1 -> Selector3/1
  Bias1/1 -> Selector4/2, Selector3/2
  Constant8/1 -> Selector4/1
  Selector3/1 -> Mux1/1
  Constant7/1 -> Mod1/2
  Selector4/1 -> Mux1/2
  Mod1/1 -> Bias1/1
  Mux1/1 -> closest_point/1
  Demux1/1 -> Windowed Closest Point Locator *Feedback the location1/1(x)
  Constant2/1 -> Windowed Closest Point Locator *Feedback the location1/3(x_array)
  Constant3/1 -> Windowed Closest Point Locator *Feedback the location1/4(y_array)
  Constant1/1 -> Mod/2
  Sum/1 -> Mod/1
  Demux1/2 -> Windowed Closest Point Locator *Feedback the location1/2(y)
  Mod/1 -> Bias3/1
  xy/1 -> Demux1/1
  look_ahead_d/1 -> m->cm/1
  m->cm/1 -> Floor/1
  Floor/1 -> Sum/1
  Constant/1 -> Selector1/1
  Selector1/1 -> Mux/1
  Constant4/1 -> Selector2/1
  Mux/1 -> xy_cmd/1
  Selector2/1 -> Mux/2
  Windowed Closest Point Locator *Feedback the location1/2(distance) -> distance/1
  Bias3/1 -> Selector1/2, Selector5/2, Selector2/2
  Constant9/1 -> Selector5/1
  Selector5/1 -> heading_cmd/1
  Constant5/1 -> Windowed Closest Point Locator *Feedback the location1/5(window)
  Memory/1 -> Windowed Closest Point Locator *Feedback the location1/7(previous_location)
  Windowed Closest Point Locator *Feedback the location1/1(location) -> Sum/2, path_i/1, Memory/1, Mod1/1
